simulink model "ntnu_leg_motion_generation"  (R2022b)
settings: Solver=VariableStepAuto  StartTime=0.0  StopTime=1  MaxStep=1e-3  RelTol=1e-3  AbsTol=1e-6
settings Model: Creator=papaveneti  LastModifiedBy=papaveneti

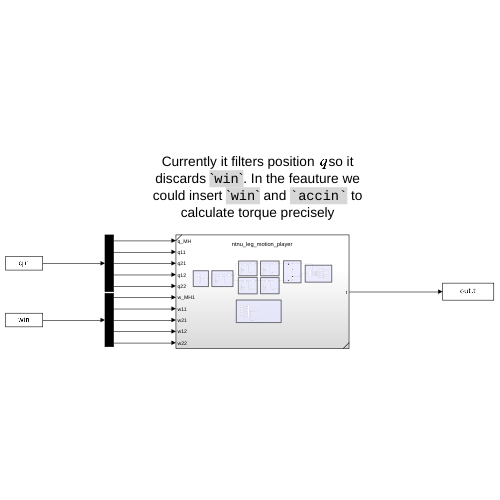
[thumbnail: Simulink's stored preview of the top-level diagram]
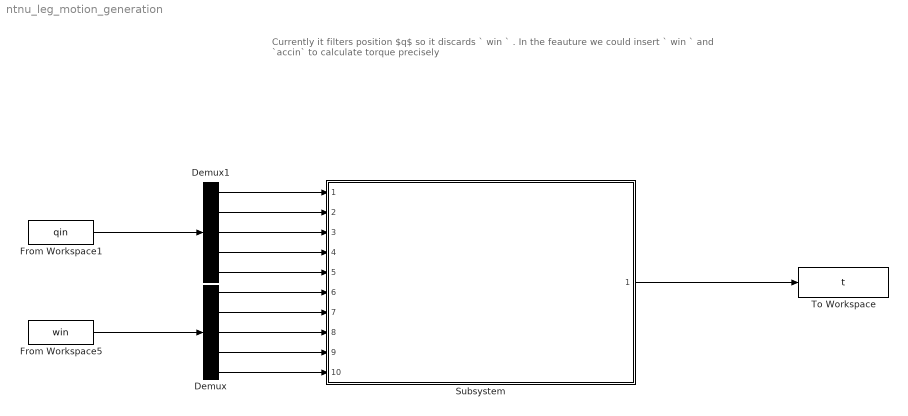
== system ntnu_leg_motion_generation ==
  note: Currently it filters position $q$ so it discards ` win ` . In the feauture we could insert ` win ` and `accin` to calculate torque precisely
  Demux : Demux  Outputs=5
  Demux1 : Demux  Outputs=5
  From Workspace1 : FromWorkspace  VariableName=qin
  From Workspace5 : FromWorkspace  VariableName=win
  Subsystem : Subsystem  ReferencedSubsystem=ntnu_leg_motion_player
  To Workspace : ToWorkspace  VariableName=t  SaveFormat=Timeseries  SampleTime=-1
  wires:
  Subsystem/1 -> To Workspace/1
  From Workspace5/1 -> Demux/1
  Demux/1 -> Subsystem/6
  Demux/2 -> Subsystem/7
  Demux/3 -> Subsystem/8
  Demux/4 -> Subsystem/9
  Demux/5 -> Subsystem/10
  From Workspace1/1 -> Demux1/1
  Demux1/1 -> Subsystem/1
  Demux1/2 -> Subsystem/2
  Demux1/3 -> Subsystem/3
  Demux1/4 -> Subsystem/4
  Demux1/5 -> Subsystem/5
